simulink model "untitled2"  (R2021b)
settings: Solver=FixedStepAuto  StartTime=0.0  StopTime=5  FixedStep=0.00005  MinStep=1e-3  RelTol=1e-3
libraries: simulink x2
settings Model: Creator=riku3  LastModifiedBy=riku3
settings SolverCC: ZeroCrossControl=DisableAll  ZeroCrossAlgorithm=Adaptive
settings DebuggingCC: IgnoredZcDiagnostic=none

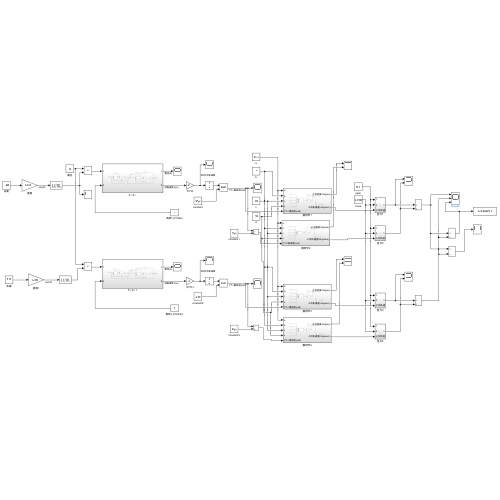
[thumbnail: Simulink's stored preview of the top-level diagram]
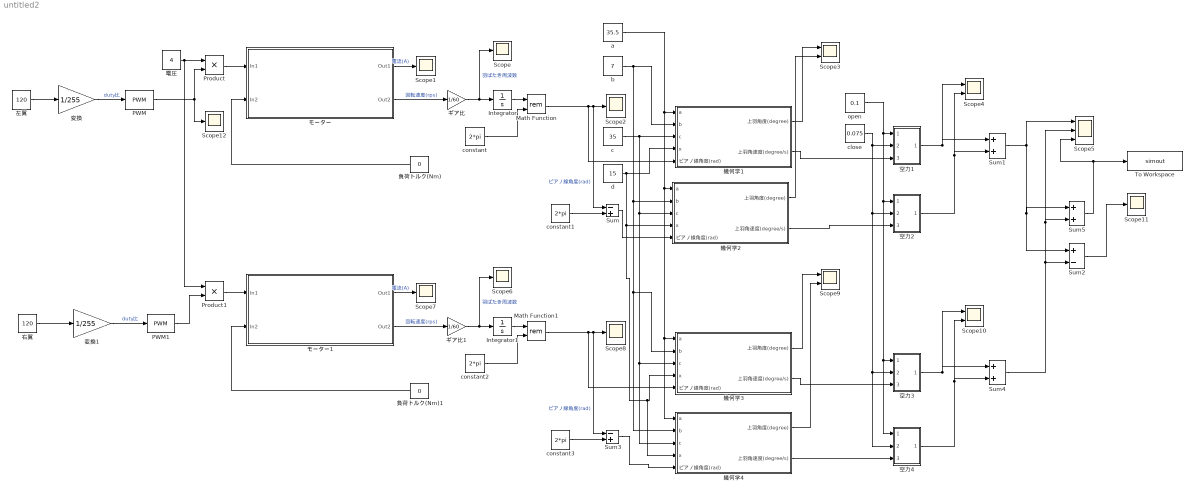
== system untitled2 ==
  Integrator : Integrator
  Integrator1 : Integrator
  Math Function : Math  Operator=rem  SaturateOnIntegerOverflow=on
  Math Function1 : Math  Operator=rem  SaturateOnIntegerOverflow=on
  PWM : simulink/Discontinuities/PWM  DisableCoverage=on  Period=0.001  DisallowZeroDutyCycle=off  RunAtFixedTimeIntervals=on  SampleTime=0.00005
  PWM1 : simulink/Discontinuities/PWM  DisableCoverage=on  Period=0.001  DisallowZeroDutyCycle=off  RunAtFixedTimeIntervals=on  SampleTime=0.00005
  Product : Product  Inputs=**
  Product1 : Product  Inputs=**
  Scope{,1..2,6..8,11..12} (8 alike) : Scope
  Scope{3..4,9..10} (4 alike) : Scope  NumInputPorts=2
  Scope5 : Scope  NumInputPorts=3
  Sum : Sum  Inputs=-+
  Sum1 : Sum  Inputs=|++
  Sum2 : Sum  Inputs=+-
  Sum3 : Sum  Inputs=-+
  Sum4 : Sum  Inputs=|++
  Sum5 : Sum  Inputs=|++
  To Workspace : ToWorkspace  VariableName=simout  SaveFormat=Timeseries  SampleTime=-1
  a : Constant  Value=35.5
  b : Constant  Value=7
  c : Constant  Value=35
  close : Constant  Value=0.075
  constant{,1..3} (4 alike) : Constant  Value=2*pi
  d : Constant  Value=15
  open : Constant  Value=0.1
  ギア比 : Gain  Gain=1/60
  ギア比1 : Gain  Gain=1/60
  モーター : Subsystem
  モーター1 : Subsystem
  右翼 : Constant  Value=120
  変換 : Gain  Gain=1/255
  変換1 : Gain  Gain=1/255
  左翼 : Constant  Value=120
  幾何学1 : Subsystem
  幾何学2 : Subsystem
  幾何学3 : Subsystem
  幾何学4 : Subsystem
  空力1 : Subsystem
  空力2 : Subsystem
  空力3 : Subsystem
  空力4 : Subsystem
  負荷トルク(Nm) : Constant  Value=0
  負荷トルク(Nm)1 : Constant  Value=0
  電圧 : Constant  Value=4
  wires:
  Sum/1 -> 幾何学2/5(ピアノ線角度(rad))
  幾何学1/1(上羽角度(degree)) -> Scope3/1
  電圧/1 -> Product/1, Product1/1
  ギア比/1 -> Integrator/1, Scope/1  "羽ばたき周波数"
  Integrator/1 -> Math Function/1
  constant/1 -> Math Function/2
  constant1/1 -> Sum/2
  モーター/1(Out1) -> Scope1/1  "電流(A)"
  負荷トルク(Nm)/1 -> モーター/2(In2)
  Product/1 -> モーター/1(In1)
  Math Function/1 -> 幾何学1/5(ピアノ線角度(rad)), Sum/1, Scope2/1  "ピアノ線角度(rad)"
  モーター/2(Out2) -> ギア比/1  "回転速度(rps)"
  空力1/1(Out1) -> Sum1/1, Scope4/1
  空力2/1(Out1) -> Sum1/2, Scope4/2
  Sum1/1 -> Sum2/1, Sum5/1, Scope5/1
  close/1 -> 空力4/2(In2), 空力3/2(In2), 空力2/2(In2), 空力1/2(In2)
  open/1 -> 空力4/1(In1), 空力3/1(In1), 空力2/1(In1), 空力1/1(In1)
  a/1 -> 幾何学2/1(a), 幾何学4/1(a), 幾何学3/1(a), 幾何学1/1(a)
  空力3/1(Out1) -> Sum4/1, Scope10/1
  Integrator1/1 -> Math Function1/1
  c/1 -> 幾何学2/3(c), 幾何学4/3(c), 幾何学3/3(c), 幾何学1/3(c)
  幾何学3/1(上羽角度(degree)) -> Scope9/1
  Math Function1/1 -> 幾何学3/5(ピアノ線角度(rad)), Sum3/1, Scope8/1  "ピアノ線角度(rad)"
  Sum3/1 -> 幾何学4/5(ピアノ線角度(rad))
  幾何学4/1(上羽角度(degree)) -> Scope9/2
  b/1 -> 幾何学2/2(b), 幾何学4/2(b), 幾何学3/2(b), 幾何学1/2(b)
  d/1 -> 幾何学1/4(x), 幾何学2/4(x), 幾何学4/4(x), 幾何学3/4(x)
  モーター1/1(Out1) -> Scope7/1  "電流(A)"
  Product1/1 -> モーター1/1(In1)
  空力4/1(Out1) -> Scope10/2, Sum4/2
  constant2/1 -> Math Function1/2
  モーター1/2(Out2) -> ギア比1/1  "回転速度(rps)"
  ギア比1/1 -> Integrator1/1, Scope6/1  "羽ばたき周波数"
  constant3/1 -> Sum3/2
  負荷トルク(Nm)1/1 -> モーター1/2(In2)
  Sum4/1 -> Sum2/2, Sum5/2, Scope5/2
  Sum2/1 -> Scope11/1
  Sum5/1 -> To Workspace/1, Scope5/3
  PWM/1 -> Scope12/1, Product/2
  PWM1/1 -> Product1/2
  変換/1 -> PWM/1  "duty比"
  左翼/1 -> 変換/1
  右翼/1 -> 変換1/1
  変換1/1 -> PWM1/1  "duty比"
  幾何学1/2(上羽角速度(degree/s)) -> 空力1/3(上羽角速度(degree/s))
  幾何学2/1(上羽角度(degree)) -> Scope3/2
  幾何学2/2(上羽角速度(degree/s)) -> 空力2/3(上羽角度(degree))
  幾何学3/2(上羽角速度(degree/s)) -> 空力3/3(上羽角速度(degree/s))
  幾何学4/2(上羽角速度(degree/s)) -> 空力4/3(上羽角度(degree))

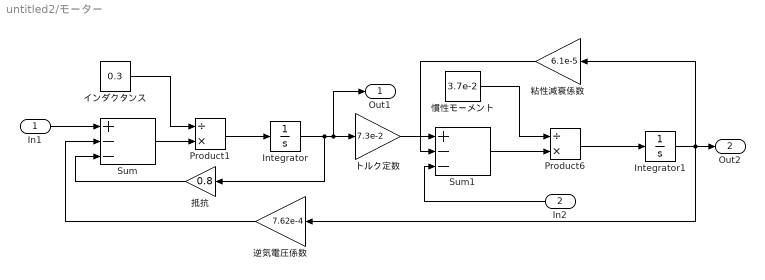
== system untitled2/モーター ==
  In1 : Inport
  In2 : Inport  Port=2
  Integrator : Integrator
  Integrator1 : Integrator  InitialCondition=600
  Product1 : Product  Inputs=/*
  Product6 : Product  Inputs=/*
  Sum : Sum  Inputs=+--
  Sum1 : Sum  Inputs=+--
  インダクタンス : Constant  Value=0.3
  トルク定数 : Gain  Gain=7.3e-2
  慣性モーメント : Constant  Value=3.7e-2
  抵抗 : Gain  Gain=0.8
  粘性減衰係数 : Gain  Gain=6.1e-5
  逆気電圧係数 : Gain  Gain=7.62e-4
  Out1 : Outport
  Out2 : Outport  Port=2
  wires:
  慣性モーメント/1 -> Product6/1
  トルク定数/1 -> Sum1/1
  粘性減衰係数/1 -> Sum1/2
  In2/1 -> Sum1/3
  抵抗/1 -> Sum/3
  逆気電圧係数/1 -> Sum/2
  In1/1 -> Sum/1
  Sum1/1 -> Product6/2
  Product1/1 -> Integrator/1
  インダクタンス/1 -> Product1/1
  Sum/1 -> Product1/2
  Product6/1 -> Integrator1/1
  Integrator1/1 -> 逆気電圧係数/1, 粘性減衰係数/1, Out2/1
  Integrator/1 -> Out1/1, トルク定数/1, 抵抗/1

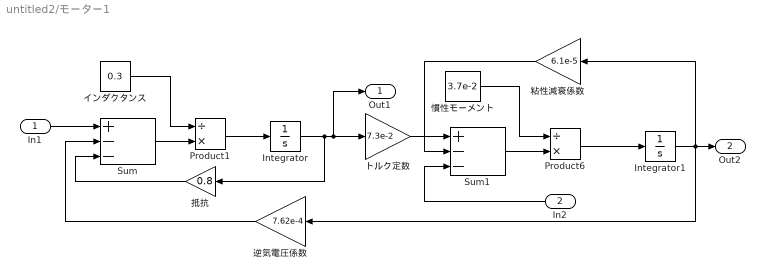
== system untitled2/モーター1 ==
  In1 : Inport
  In2 : Inport  Port=2
  Integrator : Integrator
  Integrator1 : Integrator  InitialCondition=600
  Product1 : Product  Inputs=/*
  Product6 : Product  Inputs=/*
  Sum : Sum  Inputs=+--
  Sum1 : Sum  Inputs=+--
  インダクタンス : Constant  Value=0.3
  トルク定数 : Gain  Gain=7.3e-2
  慣性モーメント : Constant  Value=3.7e-2
  抵抗 : Gain  Gain=0.8
  粘性減衰係数 : Gain  Gain=6.1e-5
  逆気電圧係数 : Gain  Gain=7.62e-4
  Out1 : Outport
  Out2 : Outport  Port=2
  wires:
  慣性モーメント/1 -> Product6/1
  トルク定数/1 -> Sum1/1
  粘性減衰係数/1 -> Sum1/2
  In2/1 -> Sum1/3
  抵抗/1 -> Sum/3
  逆気電圧係数/1 -> Sum/2
  In1/1 -> Sum/1
  Sum1/1 -> Product6/2
  Product1/1 -> Integrator/1
  インダクタンス/1 -> Product1/1
  Sum/1 -> Product1/2
  Product6/1 -> Integrator1/1
  Integrator1/1 -> 逆気電圧係数/1, 粘性減衰係数/1, Out2/1
  Integrator/1 -> Out1/1, トルク定数/1, 抵抗/1

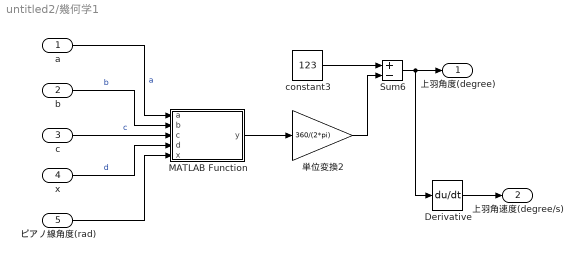
== system untitled2/幾何学1 ==
  a : Inport
  b : Inport  Port=2
  c : Inport  Port=3
  x : Inport  Port=4
  ピアノ線角度(rad) : Inport  Port=5
  Derivative : Derivative
  MATLAB Function : MATLAB Function  TreatAsAtomicUnit=on
  Sum6 : Sum  Inputs=+-
  constant3 : Constant  Value=123
  単位変換2 : Gain  Gain=360/(2*pi)
  上羽角度(degree) : Outport
  上羽角速度(degree/s) : Outport  Port=2
  wires:
  MATLAB Function/1(y) -> 単位変換2/1
  Sum6/1 -> Derivative/1, 上羽角度(degree)/1
  単位変換2/1 -> Sum6/2
  a/1 -> MATLAB Function/1(a)  "a"
  c/1 -> MATLAB Function/3(c)  "c"
  constant3/1 -> Sum6/1
  x/1 -> MATLAB Function/4(d)  "d"
  b/1 -> MATLAB Function/2(b)  "b"
  ピアノ線角度(rad)/1 -> MATLAB Function/5(x)
  Derivative/1 -> 上羽角速度(degree/s)/1

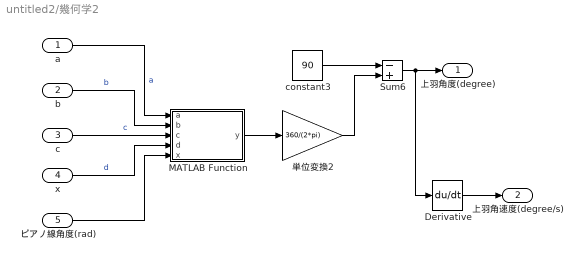
== system untitled2/幾何学2 ==
  a : Inport
  b : Inport  Port=2
  c : Inport  Port=3
  x : Inport  Port=4
  ピアノ線角度(rad) : Inport  Port=5
  Derivative : Derivative
  MATLAB Function : MATLAB Function  TreatAsAtomicUnit=on
  Sum6 : Sum  Inputs=-+
  constant3 : Constant  Value=90
  単位変換2 : Gain  Gain=360/(2*pi)
  上羽角度(degree) : Outport
  上羽角速度(degree/s) : Outport  Port=2
  wires:
  MATLAB Function/1(y) -> 単位変換2/1
  Sum6/1 -> Derivative/1, 上羽角度(degree)/1
  単位変換2/1 -> Sum6/2
  a/1 -> MATLAB Function/1(a)  "a"
  c/1 -> MATLAB Function/3(c)  "c"
  constant3/1 -> Sum6/1
  x/1 -> MATLAB Function/4(d)  "d"
  b/1 -> MATLAB Function/2(b)  "b"
  ピアノ線角度(rad)/1 -> MATLAB Function/5(x)
  Derivative/1 -> 上羽角速度(degree/s)/1

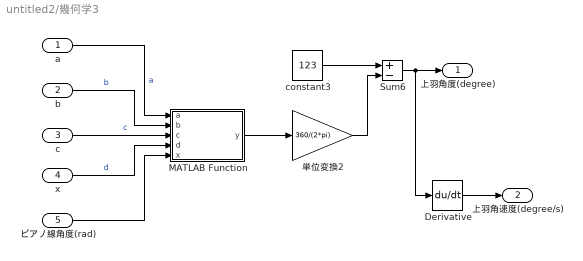
== system untitled2/幾何学3 ==
  a : Inport
  b : Inport  Port=2
  c : Inport  Port=3
  x : Inport  Port=4
  ピアノ線角度(rad) : Inport  Port=5
  Derivative : Derivative
  MATLAB Function : MATLAB Function  TreatAsAtomicUnit=on
  Sum6 : Sum  Inputs=+-
  constant3 : Constant  Value=123
  単位変換2 : Gain  Gain=360/(2*pi)
  上羽角度(degree) : Outport
  上羽角速度(degree/s) : Outport  Port=2
  wires:
  MATLAB Function/1(y) -> 単位変換2/1
  Sum6/1 -> Derivative/1, 上羽角度(degree)/1
  単位変換2/1 -> Sum6/2
  a/1 -> MATLAB Function/1(a)  "a"
  c/1 -> MATLAB Function/3(c)  "c"
  constant3/1 -> Sum6/1
  x/1 -> MATLAB Function/4(d)  "d"
  b/1 -> MATLAB Function/2(b)  "b"
  ピアノ線角度(rad)/1 -> MATLAB Function/5(x)
  Derivative/1 -> 上羽角速度(degree/s)/1

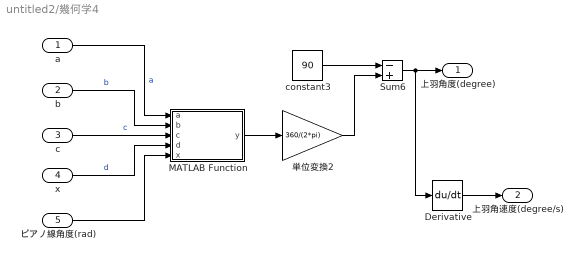
== system untitled2/幾何学4 ==
  a : Inport
  b : Inport  Port=2
  c : Inport  Port=3
  x : Inport  Port=4
  ピアノ線角度(rad) : Inport  Port=5
  Derivative : Derivative
  MATLAB Function : MATLAB Function  TreatAsAtomicUnit=on
  Sum6 : Sum  Inputs=-+
  constant3 : Constant  Value=90
  単位変換2 : Gain  Gain=360/(2*pi)
  上羽角度(degree) : Outport
  上羽角速度(degree/s) : Outport  Port=2
  wires:
  MATLAB Function/1(y) -> 単位変換2/1
  Sum6/1 -> Derivative/1, 上羽角度(degree)/1
  単位変換2/1 -> Sum6/2
  a/1 -> MATLAB Function/1(a)  "a"
  c/1 -> MATLAB Function/3(c)  "c"
  constant3/1 -> Sum6/1
  x/1 -> MATLAB Function/4(d)  "d"
  b/1 -> MATLAB Function/2(b)  "b"
  ピアノ線角度(rad)/1 -> MATLAB Function/5(x)
  Derivative/1 -> 上羽角速度(degree/s)/1

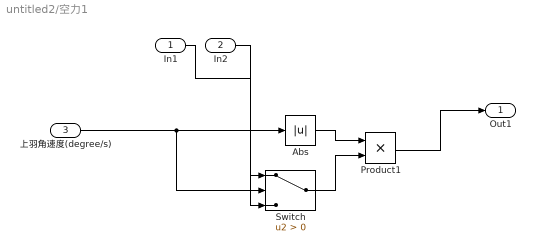
== system untitled2/空力1 ==
  In1 : Inport
  In2 : Inport  Port=2
  上羽角速度(degree/s) : Inport  Port=3
  Abs : Abs
  Product1 : Product
  Switch : Switch  Criteria=u2 > Threshold
  Out1 : Outport
  wires:
  Abs/1 -> Product1/1
  Switch/1 -> Product1/2
  Product1/1 -> Out1/1
  In1/1 -> Switch/1
  In2/1 -> Switch/3
  上羽角速度(degree/s)/1 -> Switch/2, Abs/1

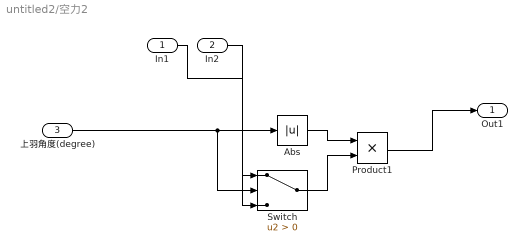
== system untitled2/空力2 ==
  In1 : Inport
  In2 : Inport  Port=2
  上羽角度(degree) : Inport  Port=3
  Abs : Abs
  Product1 : Product
  Switch : Switch  Criteria=u2 > Threshold
  Out1 : Outport
  wires:
  Abs/1 -> Product1/1
  Switch/1 -> Product1/2
  Product1/1 -> Out1/1
  In1/1 -> Switch/1
  上羽角度(degree)/1 -> Switch/2, Abs/1
  In2/1 -> Switch/3

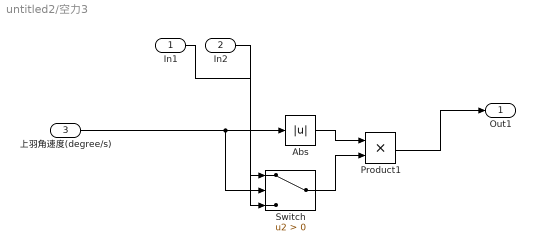
== system untitled2/空力3 ==
  In1 : Inport
  In2 : Inport  Port=2
  上羽角速度(degree/s) : Inport  Port=3
  Abs : Abs
  Product1 : Product
  Switch : Switch  Criteria=u2 > Threshold
  Out1 : Outport
  wires:
  Abs/1 -> Product1/1
  Switch/1 -> Product1/2
  Product1/1 -> Out1/1
  In1/1 -> Switch/1
  上羽角速度(degree/s)/1 -> Switch/2, Abs/1
  In2/1 -> Switch/3

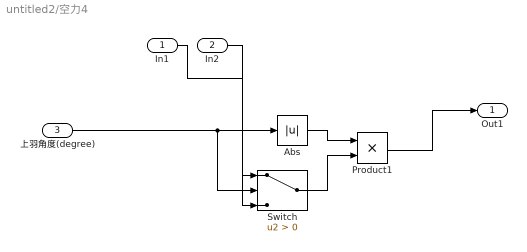
== system untitled2/空力4 ==
  In1 : Inport
  In2 : Inport  Port=2
  上羽角度(degree) : Inport  Port=3
  Abs : Abs
  Product1 : Product
  Switch : Switch  Criteria=u2 > Threshold
  Out1 : Outport
  wires:
  Abs/1 -> Product1/1
  Switch/1 -> Product1/2
  Product1/1 -> Out1/1
  In1/1 -> Switch/1
  上羽角度(degree)/1 -> Switch/2, Abs/1
  In2/1 -> Switch/3

== matlab function untitled2/幾何学2/MATLAB Function ==
  data: a input; y output; b input; c input; d input; x input
function y = fcn(a,b,c,d,x)

h2 = a^2+b^2+2*a*b*cos(x);
h = sqrt(h2);
p = acos((h2+a^2-b^2)/(2*h*a));
q = acos((h2+d^2-c^2)/(2*h*d));

if x>pi()
    p = -1*p;
    y = p+q;
else
    y = p+q;
end

== matlab function untitled2/幾何学1/MATLAB Function ==
  data: a input; y output; b input; c input; d input; x input
function y = fcn(a,b,c,d,x)

h2 = a^2+b^2+2*a*b*cos(x);
h = sqrt(h2);
p = acos((h2+a^2-b^2)/(2*h*a));
q = acos((h2+d^2-c^2)/(2*h*d));

if x>pi()
    p = -1*p;
    y = p+q;
else
    y = p+q;
end

== matlab function untitled2/幾何学3/MATLAB Function ==
  data: a input; y output; b input; c input; d input; x input
function y = fcn(a,b,c,d,x)

h2 = a^2+b^2+2*a*b*cos(x);
h = sqrt(h2);
p = acos((h2+a^2-b^2)/(2*h*a));
q = acos((h2+d^2-c^2)/(2*h*d));

if x>pi()
    p = -1*p;
    y = p+q;
else
    y = p+q;
end

== matlab function untitled2/幾何学4/MATLAB Function ==
  data: a input; y output; b input; c input; d input; x input
function y = fcn(a,b,c,d,x)

h2 = a^2+b^2+2*a*b*cos(x);
h = sqrt(h2);
p = acos((h2+a^2-b^2)/(2*h*a));
q = acos((h2+d^2-c^2)/(2*h*d));

if x>pi()
    p = -1*p;
    y = p+q;
else
    y = p+q;
end
